simulink model "Full_Model_R1"  (R2013a)
settings: Solver=ode45  StartTime=0.0  StopTime=10.0  RelTol=1e-3
undefined symbols (not defined in the file or in its folder): B, D, g, I_Phi, I_Theta, I_Yaw, J, Kf, Kw, L, Mass, MotorTau
settings Model: Creator=Ross  LastModifiedBy=Ross

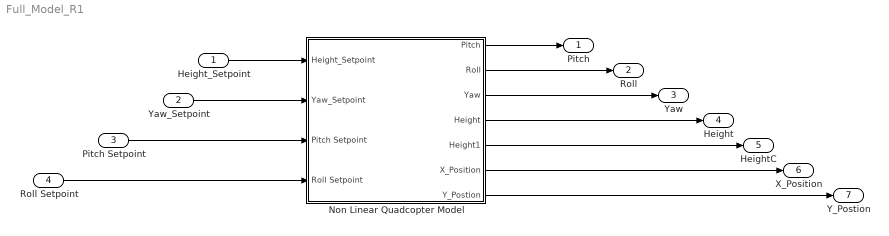
== system Full_Model_R1 ==
  Height_Setpoint : Inport
  Yaw_Setpoint : Inport  Port=2
  Pitch Setpoint : Inport  Port=3
  Roll Setpoint : Inport  Port=4
  Non Linear Quadcopter Model : Subsystem
  Pitch : Outport
  Roll : Outport  Port=2
  Yaw : Outport  Port=3
  Height : Outport  Port=4
  HeightC : Outport  Port=5
  X_Position : Outport  Port=6
  Y_Postion : Outport  Port=7
  wires:
  Height_Setpoint/1 -> Non Linear Quadcopter Model/1(Height_Setpoint)
  Yaw_Setpoint/1 -> Non Linear Quadcopter Model/2(Yaw_Setpoint)
  Pitch Setpoint/1 -> Non Linear Quadcopter Model/3(Pitch Setpoint)
  Roll Setpoint/1 -> Non Linear Quadcopter Model/4(Roll Setpoint)
  Non Linear Quadcopter Model/1(Pitch) -> Pitch/1
  Non Linear Quadcopter Model/2(Roll) -> Roll/1
  Non Linear Quadcopter Model/3(Yaw) -> Yaw/1
  Non Linear Quadcopter Model/4(Height) -> Height/1
  Non Linear Quadcopter Model/5(Height1) -> HeightC/1
  Non Linear Quadcopter Model/6(X_Position) -> X_Position/1
  Non Linear Quadcopter Model/7(Y_Postion) -> Y_Postion/1

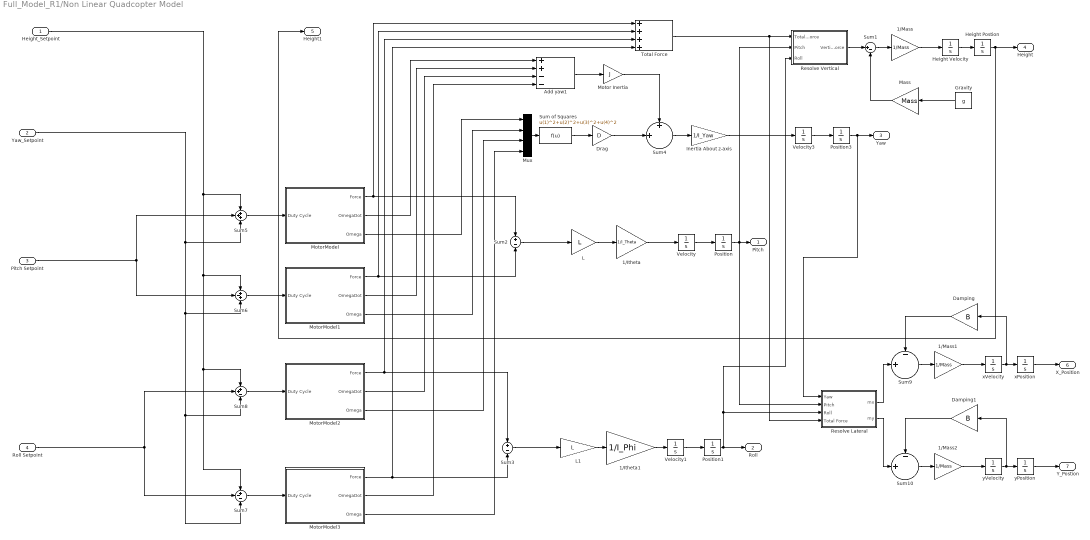
== system Full_Model_R1/Non Linear Quadcopter Model ==
  Height_Setpoint : Inport
  Yaw_Setpoint : Inport  Port=2
  Pitch Setpoint : Inport  Port=3
  Roll Setpoint : Inport  Port=4
  1/Itheta : Gain  Gain=1/I_Theta
  1/Itheta1 : Gain  Gain=1/I_Phi
  1/Mass : Gain  Gain=1/Mass
  1/Mass1 : Gain  Gain=1/Mass
  1/Mass2 : Gain  Gain=1/Mass
  Add yaw1 : Sum  Inputs=++--
  Damping : Gain  Gain=B
  Damping1 : Gain  Gain=B
  Drag : Gain  Gain=D
  Gravity : Constant  Value=g
  Height Postion : Integrator
  Height Velocity : Integrator
  Inertia About z-axis : Gain  Gain=1/I_Yaw
  L : Gain  Gain=L
  L1 : Gain  Gain=L
  Mass : Gain  Gain=Mass
  Motor Inertia : Gain  Gain=J
  MotorModel : Subsystem
  MotorModel1 : Subsystem
  MotorModel2 : Subsystem
  MotorModel3 : Subsystem
  Mux : Mux
  Position : Integrator
  Position1 : Integrator
  Position3 : Integrator
  Resolve Lateral : Subsystem
  Resolve Vertical : Subsystem
  Sum of Squares : Fcn  Expr=u(1)^2+u(2)^2+u(3)^2+u(4)^2
  Sum1 : Sum  Inputs=|+-
  Sum10 : Sum  Inputs=-|||+||||
  Sum2 : Sum  Inputs=+|-
  Sum3 : Sum  Inputs=+|-
  Sum4 : Sum  Inputs=+|||+||||
  Sum5 : Sum  Inputs=+++
  Sum6 : Sum  Inputs=+-+
  Sum7 : Sum  Inputs=+--
  Sum8 : Sum  Inputs=++-
  Sum9 : Sum  Inputs=-|||+||||
  Total Force : Sum  Inputs=++++
  Velocity : Integrator
  Velocity1 : Integrator
  Velocity3 : Integrator
  xPosition : Integrator
  xVelocity : Integrator
  yPosition : Integrator
  yVelocity : Integrator
  Pitch : Outport
  Roll : Outport  Port=2
  Yaw : Outport  Port=3
  Height : Outport  Port=4
  Height1 : Outport  Port=5
  X_Position : Outport  Port=6
  Y_Postion : Outport  Port=7
  wires:
  Sum1/1 -> 1/Mass/1
  Pitch Setpoint/1 -> Sum6/2, Sum5/2
  Add yaw1/1 -> Motor Inertia/1
  Mass/1 -> Sum1/2
  1/Mass/1 -> Height Velocity/1
  Motor Inertia/1 -> Sum4/1
  1/Mass1/1 -> xVelocity/1
  Sum9/1 -> 1/Mass1/1
  xPosition/1 -> X_Position/1
  Damping/1 -> Sum9/1
  xVelocity/1 -> Damping/1, xPosition/1
  MotorModel/2(OmegaDot) -> Add yaw1/1
  Sum8/1 -> MotorModel2/1(Duty Cycle)
  Height Velocity/1 -> Height Postion/1
  L/1 -> 1/Itheta/1
  1/Itheta/1 -> Velocity/1
  Sum2/1 -> L/1
  Velocity/1 -> Position/1
  Position/1 -> Pitch/1, Resolve Lateral/2(Pitch), Resolve Vertical/2(Pitch)
  Total Force/1 -> Resolve Lateral/4(Total Force), Resolve Vertical/1(Total Force)
  Sum of Squares/1 -> Drag/1
  Drag/1 -> Sum4/2
  Position3/1 -> Yaw/1, Resolve Lateral/1(Yaw)
  Velocity3/1 -> Position3/1
  Inertia About z-axis/1 -> Velocity3/1
  MotorModel3/1(Force) -> Total Force/4, Sum3/2
  L1/1 -> 1/Itheta1/1
  Velocity1/1 -> Position1/1
  Sum3/1 -> L1/1
  Position1/1 -> Roll/1, Resolve Lateral/3(Roll), Resolve Vertical/3(Roll)
  1/Itheta1/1 -> Velocity1/1
  Resolve Vertical/1(Vertical Force) -> Sum1/1
  MotorModel/1(Force) -> Sum2/1, Total Force/1
  Sum10/1 -> 1/Mass2/1
  1/Mass2/1 -> yVelocity/1
  yPosition/1 -> Y_Postion/1
  Damping1/1 -> Sum10/1
  yVelocity/1 -> Damping1/1, yPosition/1
  Height Postion/1 -> Height1/1, Height/1
  Sum7/1 -> MotorModel3/1(Duty Cycle)
  Sum6/1 -> MotorModel1/1(Duty Cycle)
  MotorModel2/2(OmegaDot) -> Add yaw1/3
  MotorModel1/1(Force) -> Sum2/2, Total Force/2
  Sum4/1 -> Inertia About z-axis/1
  MotorModel2/1(Force) -> Sum3/1, Total Force/3
  Height_Setpoint/1 -> Sum6/1, Sum7/1, Sum8/1, Sum5/1
  Yaw_Setpoint/1 -> Sum7/3, Sum8/3, Sum6/3, Sum5/3
  MotorModel1/2(OmegaDot) -> Add yaw1/2
  MotorModel3/2(OmegaDot) -> Add yaw1/4
  Sum5/1 -> MotorModel/1(Duty Cycle)
  Roll Setpoint/1 -> Sum8/2, Sum7/2
  Gravity/1 -> Mass/1
  Resolve Lateral/1(mx) -> Sum9/2
  Resolve Lateral/2(my) -> Sum10/2
  MotorModel/3(Omega) -> Mux/1
  MotorModel1/3(Omega) -> Mux/2
  MotorModel2/3(Omega) -> Mux/3
  MotorModel3/3(Omega) -> Mux/4
  Mux/1 -> Sum of Squares/1

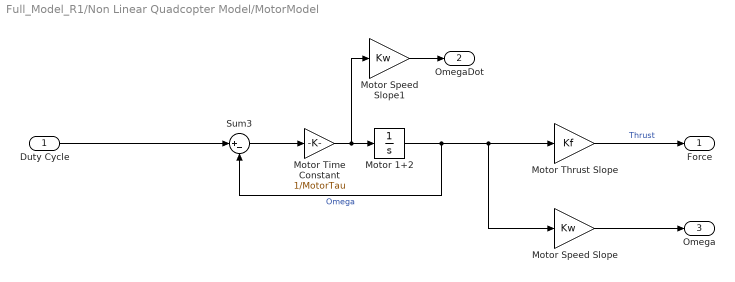
== system Full_Model_R1/Non Linear Quadcopter Model/MotorModel ==
  Duty Cycle : Inport
  Motor 1+2 : Integrator
  Motor Speed Slope : Gain  Gain=Kw
  Motor Speed Slope1 : Gain  Gain=Kw
  Motor Thrust Slope : Gain  Gain=Kf
  Motor Time Constant : Gain  Gain=1/MotorTau
  Sum3 : Sum  Inputs=|+-
  Force : Outport
  OmegaDot : Outport  Port=2
  Omega : Outport  Port=3
  wires:
  Motor Thrust Slope/1 -> Force/1  "Thrust"
  Motor 1+2/1 -> Sum3/2, Motor Speed Slope/1, Motor Thrust Slope/1  "Omega"
  Duty Cycle/1 -> Sum3/1
  Sum3/1 -> Motor Time Constant/1
  Motor Time Constant/1 -> Motor 1+2/1, Motor Speed Slope1/1
  Motor Speed Slope/1 -> Omega/1
  Motor Speed Slope1/1 -> OmegaDot/1

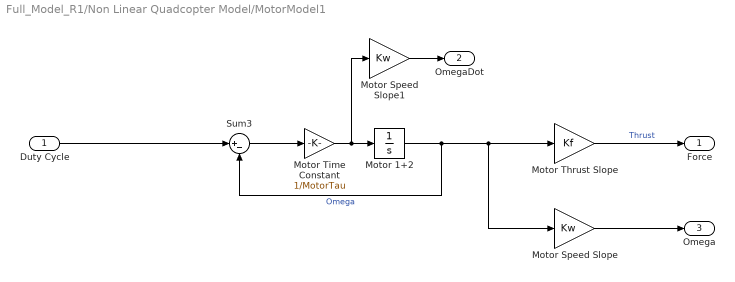
== system Full_Model_R1/Non Linear Quadcopter Model/MotorModel1 ==
  Duty Cycle : Inport
  Motor 1+2 : Integrator
  Motor Speed Slope : Gain  Gain=Kw
  Motor Speed Slope1 : Gain  Gain=Kw
  Motor Thrust Slope : Gain  Gain=Kf
  Motor Time Constant : Gain  Gain=1/MotorTau
  Sum3 : Sum  Inputs=|+-
  Force : Outport
  OmegaDot : Outport  Port=2
  Omega : Outport  Port=3
  wires:
  Motor Thrust Slope/1 -> Force/1  "Thrust"
  Motor 1+2/1 -> Sum3/2, Motor Speed Slope/1, Motor Thrust Slope/1  "Omega"
  Duty Cycle/1 -> Sum3/1
  Sum3/1 -> Motor Time Constant/1
  Motor Time Constant/1 -> Motor 1+2/1, Motor Speed Slope1/1
  Motor Speed Slope/1 -> Omega/1
  Motor Speed Slope1/1 -> OmegaDot/1

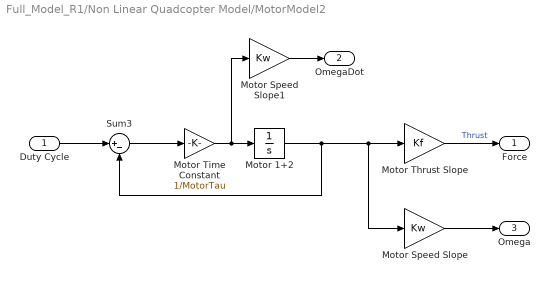
== system Full_Model_R1/Non Linear Quadcopter Model/MotorModel2 ==
  Duty Cycle : Inport
  Motor 1+2 : Integrator
  Motor Speed Slope : Gain  Gain=Kw
  Motor Speed Slope1 : Gain  Gain=Kw
  Motor Thrust Slope : Gain  Gain=Kf
  Motor Time Constant : Gain  Gain=1/MotorTau
  Sum3 : Sum  Inputs=|+-
  Force : Outport
  OmegaDot : Outport  Port=2
  Omega : Outport  Port=3
  wires:
  Motor Thrust Slope/1 -> Force/1  "Thrust"
  Motor 1+2/1 -> Sum3/2, Motor Speed Slope/1, Motor Thrust Slope/1
  Duty Cycle/1 -> Sum3/1
  Sum3/1 -> Motor Time Constant/1
  Motor Time Constant/1 -> Motor 1+2/1, Motor Speed Slope1/1
  Motor Speed Slope/1 -> Omega/1
  Motor Speed Slope1/1 -> OmegaDot/1

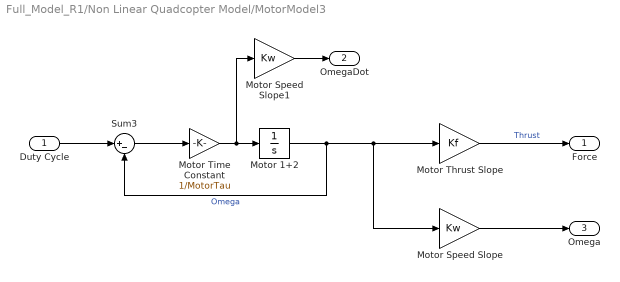
== system Full_Model_R1/Non Linear Quadcopter Model/MotorModel3 ==
  Duty Cycle : Inport
  Motor 1+2 : Integrator
  Motor Speed Slope : Gain  Gain=Kw
  Motor Speed Slope1 : Gain  Gain=Kw
  Motor Thrust Slope : Gain  Gain=Kf
  Motor Time Constant : Gain  Gain=1/MotorTau
  Sum3 : Sum  Inputs=|+-
  Force : Outport
  OmegaDot : Outport  Port=2
  Omega : Outport  Port=3
  wires:
  Motor Thrust Slope/1 -> Force/1  "Thrust"
  Motor 1+2/1 -> Sum3/2, Motor Speed Slope/1, Motor Thrust Slope/1  "Omega"
  Duty Cycle/1 -> Sum3/1
  Sum3/1 -> Motor Time Constant/1
  Motor Time Constant/1 -> Motor 1+2/1, Motor Speed Slope1/1
  Motor Speed Slope/1 -> Omega/1
  Motor Speed Slope1/1 -> OmegaDot/1

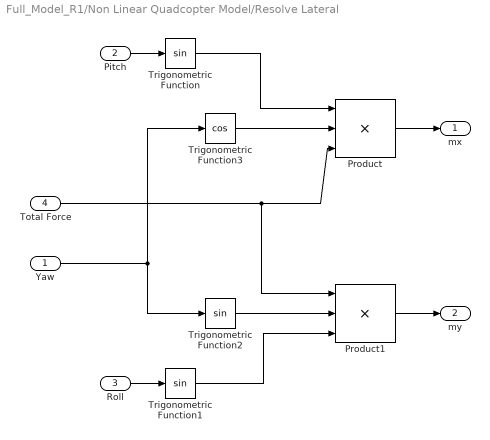
== system Full_Model_R1/Non Linear Quadcopter Model/Resolve Lateral ==
  Yaw : Inport
  Pitch : Inport  Port=2
  Roll : Inport  Port=3
  Total Force : Inport  Port=4
  Product : Product  Inputs=3
  Product1 : Product  Inputs=3
  Trigonometric Function : Trigonometry
  Trigonometric Function1 : Trigonometry
  Trigonometric Function2 : Trigonometry
  Trigonometric Function3 : Trigonometry  Operator=cos
  mx : Outport
  my : Outport  Port=2
  wires:
  Trigonometric Function/1 -> Product/1
  Total Force/1 -> Product1/1, Product/3
  Product/1 -> mx/1
  Roll/1 -> Trigonometric Function1/1
  Trigonometric Function1/1 -> Product1/3
  Product1/1 -> my/1
  Trigonometric Function3/1 -> Product/2
  Trigonometric Function2/1 -> Product1/2
  Yaw/1 -> Trigonometric Function2/1, Trigonometric Function3/1
  Pitch/1 -> Trigonometric Function/1

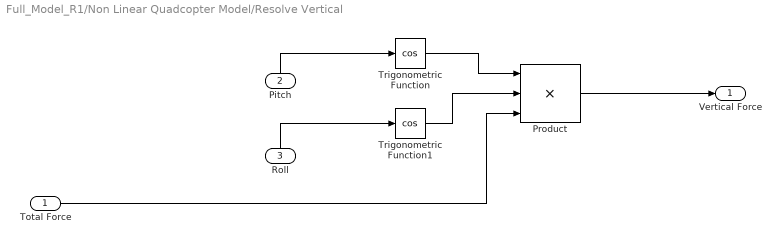
== system Full_Model_R1/Non Linear Quadcopter Model/Resolve Vertical ==
  Total Force : Inport
  Pitch : Inport  Port=2
  Roll : Inport  Port=3
  Product : Product  Inputs=3
  Trigonometric Function : Trigonometry  Operator=cos
  Trigonometric Function1 : Trigonometry  Operator=cos
  Vertical Force : Outport
  wires:
  Trigonometric Function/1 -> Product/1
  Total Force/1 -> Product/3
  Roll/1 -> Trigonometric Function1/1
  Pitch/1 -> Trigonometric Function/1
  Product/1 -> Vertical Force/1
  Trigonometric Function1/1 -> Product/2
